simulink model "CameraExample_2"  (R2016a)
settings: Solver=FixedStepDiscrete  StartTime=0.0  StopTime=inf  RelTol=1e-3
libraries: matlabGenericSHM_Block x2
settings Model: Creator=aurora  LastModifiedBy=migf1
settings DataIOCC: SaveFormat=Array  SaveOutput=off  SaveTime=off
settings OptimizationCC: SimCompilerOptimization=on
settings DebuggingCC: SolverPrmCheckMsg=warning
settings HardwareCC: ProdBitPerPointer=32  ProdLargestAtomicFloat=None  ProdIntDivRoundTo=Undefined  ProdEndianess=Unspecified  ProdWordSize=32  ProdHWDeviceType=32-bit Generic
settings ModelReferenceCC: PropagateSignalLabelsOutOfModel=off
settings ConfigComp: CovModelRefEnable=Off  CovSFcnEnable=off

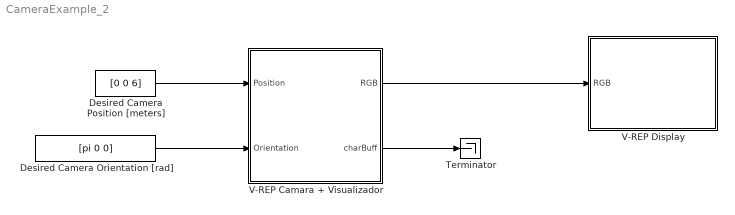
== system CameraExample_2 ==
  Desired Camera Orientation [rad] : Constant  Value=[pi 0 0]  OutDataTypeStr=single
  Desired Camera Position [meters] : Constant  Value=[0 0 6]  OutDataTypeStr=single
  Terminator : Terminator
  V-REP Camara + Visualizador : Subsystem  mask{ResX=512, ResY=512, id=4}
      mask prompts: ResX "Camera  X resolution"; ResY "Camera Y resolution"; id "Share Memory Id"
      mask Display:
      | image('webcam.jpg')
      | color('red');
      | port_label('input',1,'Position')
      | port_label('input',2,'Orientation')
      | port_label('output',1,'RGB')
      | port_label('output',2,'Char Buffer')
  V-REP Display : Subsystem  mask{ResX=512, ResY=512, id=11}
      mask prompts: ResX "Display X resolution"; ResY "Display Y resolution"; id "Share Memory Id"
      mask Display:
      | image('display.jpg')
      | color('white');
      | port_label('input',1,'RGB')
  wires:
  V-REP Camara + Visualizador/1(RGB) -> V-REP Display/1("RGB ")
  Desired Camera Position [meters]/1 -> V-REP Camara + Visualizador/1("Position ")
  Desired Camera Orientation [rad]/1 -> V-REP Camara + Visualizador/2(Orientation)
  V-REP Camara + Visualizador/2(charBuff) -> Terminator/1

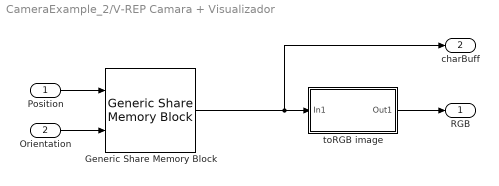
== system CameraExample_2/V-REP Camara + Visualizador ==
  "Position " : Inport
  Orientation : Inport  Port=2
  Generic Share Memory Block : matlabGenericSHM_Block/Generic Share Memory Block  nombre='vrepCam'  dispositivo=id  vecE=[3 3]  vecS=[3*ResX*ResY]  tipoE=['f' 'f']  tipoS=['C']
  toRGB image : Subsystem  mask{ResX=ResX, ResY=ResY}
      mask prompts: ResX "Resolucion Camara X"; ResY "Resolucion Camara Y"
      mask Display:
      | port_label('output', 1, 'RGB')
      | port_label('input', 1, 'videoIN')
  RGB : Outport
  charBuff : Outport  Port=2
  wires:
  Generic Share Memory Block/1 -> charBuff/1, toRGB image/1(In1)
  Orientation/1 -> Generic Share Memory Block/2
  toRGB image/1(Out1) -> RGB/1
  "Position "/1 -> Generic Share Memory Block/1

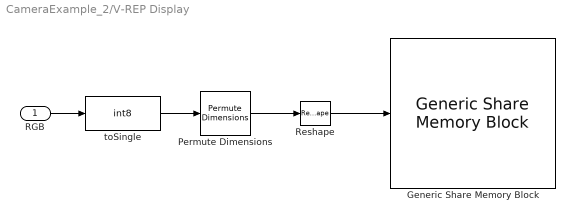
== system CameraExample_2/V-REP Display ==
  "RGB " : Inport
  Generic Share Memory Block : matlabGenericSHM_Block/Generic Share Memory Block  nombre='vrepDisplay'  dispositivo=id  vecE=[3*ResX*ResY]  vecS=[]  tipoE=['c']  tipoS=[]
  Permute Dimensions : PermuteDimensions  Order=[3,2,1]
  Reshape : Reshape
  toSingle : DataTypeConversion  OutDataTypeStr=int8
  wires:
  toSingle/1 -> Permute Dimensions/1
  "RGB "/1 -> toSingle/1
  Reshape/1 -> Generic Share Memory Block/1
  Permute Dimensions/1 -> Reshape/1

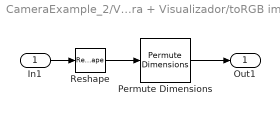
== system CameraExample_2/V-REP Camara + Visualizador/toRGB image ==
  In1 : Inport
  Permute Dimensions : PermuteDimensions  Order=[3 2 1]
  Reshape : Reshape  OutputDimensionality=Customize  OutputDimensions=[3,ResX,ResY]
  Out1 : Outport
  wires:
  Permute Dimensions/1 -> Out1/1
  Reshape/1 -> Permute Dimensions/1
  In1/1 -> Reshape/1
